simulink model "example_HeatPump"  (R2018b)
settings: Solver=ode45  StartTime=0.0  StopTime=1*24*3600  RelTol=1e-4  AbsTol=1e-5  EnableMultiTasking=on
undefined symbols (not defined in the file): path_carnot
libraries: carnot x6, simulink x1
settings Model: Creator=drhf  LastModifiedBy=P41573
settings SolverCC: AutoScaleAbsTol=off
settings DataIOCC: LimitDataPoints=on  SaveFormat=Array
settings OptimizationCC: ExpressionDepthLimit=2147483647  LifeSpan=inf
settings DebuggingCC: UnderspecifiedInitializationDetection=Classic  MergeDetectMultiDrivingBlocksExec=none  SolverPrmCheckMsg=warning  StateNameClashWarn=warning  SFUnexpectedBacktrackingDiag=warning  SFNoUnconditionalDefaultTransitionDiag=warning  SFExecutionAtInitializationDiag=none
settings HardwareCC: ProdBitPerPointer=32  ProdBitPerSizeT=32  ProdBitPerPtrDiffT=32  ProdLargestAtomicFloat=None  ProdIntDivRoundTo=Undefined  ProdEndianess=Unspecified  ProdWordSize=32  ProdHWDeviceType=32-bit Generic
settings ModelReferenceCC: PropagateSignalLabelsOutOfModel=off
settings SFSimCC: SimUseLocalCustomCode=off
settings RTWCC: RTWUseLocalCustomCode=off
settings CodeAppCC: StateflowObjectComments=on
settings GRTTargetCC: TargetLangStandard=C89/C90 (ANSI)  GeneratePreprocessorConditionals=Disable all  CombineOutputUpdateFcns=off  GRTInterface=on
settings ConfigComp: CovMetricSettings=dw  CovHtmlReporting=on  CovSaveCumulativeToWorkspaceVar=on  CovSaveSingleToWorkspaceVar=on  CovExternalEMLEnable=off

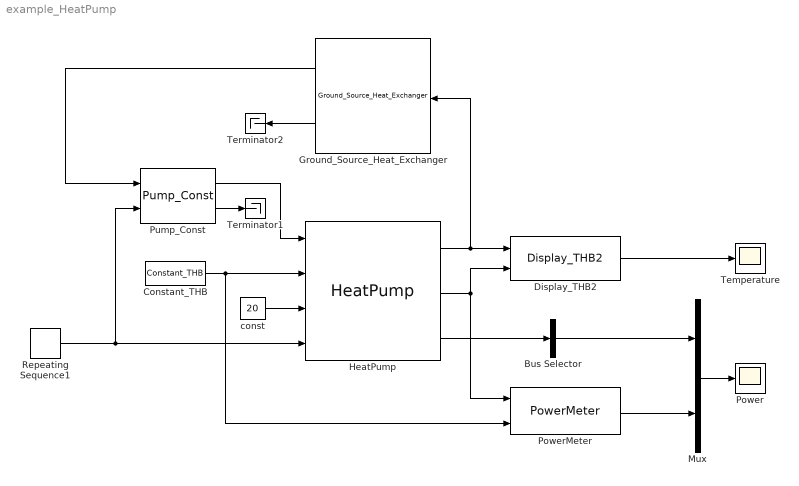
== system example_HeatPump ==
  Bus Selector : BusSelector  OutputSignals=Pelec,Qdot_cold,Qdot_hot  OutputAsBus=on
  Constant_THB : carnot/Source/Simple/Constant_THB  t=40  mdot=2000/3600  p=1e5  mID=No Pressure Drop  fluid=Water  mix=0  mix2=0  mix3=0  dia=0.02  hgt=0
  Display_THB2 : carnot/Outputs/Display_THB2  t=on  m=off  p=off  id=off  mix=off  d=off
  Ground_Source_Heat_Exchanger : carnot/Source/Heat_Pump/Ground_Source_Heat_Exchanger  Jahresmitteltemp_C=12  TGrad=0.025  lambdaErde=2.0  cpErde=800  rhoErde=2500  lambdaFill=1.0  cpFill=1000  rhoFill=2000  Sondelaenge=100  B=10  Sondendurchmesser=0.032  Bohrdurchmesser=0.18  sondenfall=2 probes B/H = 0.1  np=2  DimAxi=10  DimRad=10  Gitterfaktor=2.5
  HeatPump : carnot/Source/Heat_Pump/HeatPump  PathName=fullfile(path_carnot('libsl'), 'Source','Heat_Pump','HeatPump','parameter_set')  FileName='DefaultHeatPump.mat'  userPath=off  userParam=off  K=[299.999998982327 -59.9999988176087 12249.9999711932 -6.66666603880034 60.0000010482174 -5.13158332307255e-05 306.666667839537 -115.000000230844 12225.0000010917]  caph=32000  capc=32000  UA=6  relQdotMin=1  linc=10  quac=100  linh=10  quah=100
  Mux : Mux  Inputs=2
  Power : Scope
  PowerMeter : carnot/Control/PowerMeter
  Pump_Const : carnot/Hydraulics/Pump_Const  mdotmax=3000/3600  dia=0.0157  p0=3e5  fluid_id=Water  mix=0  mix2=0  mix3=0  UA=3  mcp=4000  Tini=20  e0=10  e1=10  e2=-1
  Repeating Sequence1 : simulink/Sources/Repeating Sequence  rep_seq_t=[0 0.5 1.5 2]*3600  rep_seq_y=[0 1 1 0]
  Temperature : Scope
  Terminator1 : Terminator
  Terminator2 : Terminator
  const : Constant  Value=20
  wires:
  Repeating Sequence1/1 -> Pump_Const/2, HeatPump/4
  Display_THB2/1 -> Temperature/1
  Mux/1 -> Power/1
  PowerMeter/1 -> Mux/2
  Bus Selector/1 -> Mux/1
  HeatPump/3 -> Bus Selector/1
  HeatPump/1 -> Ground_Source_Heat_Exchanger/1, Display_THB2/1
  HeatPump/2 -> Display_THB2/2, PowerMeter/1
  const/1 -> HeatPump/3
  Constant_THB/1 -> PowerMeter/2, HeatPump/2
  Pump_Const/1 -> HeatPump/1
  Pump_Const/2 -> Terminator1/1
  Ground_Source_Heat_Exchanger/2 -> Terminator2/1
  Ground_Source_Heat_Exchanger/1 -> Pump_Const/1
